simulink library "socmemlib"  (R2021a)
settings: Solver=VariableStepAuto  StartTime=0.0  StopTime=10.0  RelTol=1e-3
PreLoadFcn:
  | soc.internal.HWSWMessageTypeDef();
  | hsb.blkcb2.defineTypes;
undefined symbols (not defined in the file or in its folder): BurstRequest2BusObj, gcbh, hsb, m, ReadAccessBusObj, rearb, RegA, sendFifoFreeMsg, soc, WriteAccessBusObj
libraries: socmemlib_internal x59, priv_hsblib_beta2 x34, socsharedlib_internal x2, socqueuelib_internal x1, simulink x1
(part 3 of 5)

== system socmemlib/IP Core Register Read/Variant/SIM ==
  Wireless Read : socqueuelib_internal/Wireless Read  RegisterName=RegA  DataTypeStr=uint16  Dimensions=1  HoldOutput=on  SampleTime=SampleTime
      settings: SourceProductBaseCode=HW
  " Data" : Outport  VectorParamsAs1DForOutWhenUnconnected=off
  wires:
  Wireless Read/1 -> " Data"/1

== system socmemlib/Memory Channel/Reader 1/From Memory Channel ==
  "readResult " : Inport
  "ctrlIn " : Inport  Port=2
  memReady : Inport  Port=3
  Addressable From Memory Channel : Subsystem  VariantControl=AddressableFromMemory_Variant  mask{PipelineDepth=4, InterconnectDepth=ChTLASTCount}
      mask prompts: PipelineDepth "Read pipeline depth:"; InterconnectDepth "Interconnect queue depth:"
  Software Streaming From Memory Channel : Subsystem  VariantControl=SoftwareStreamingFromMemory_Variant  mask{ReadEventID=BufferEventID, ReadEventVal=[0  0  0  0  0  0  0  0  0  0  0  0  0  0  0  0  0  0  0  0  0  0  0  0  0  0  0  0  0  0  0  0  0  0  0  0  0  0  0  0  0  0  0  0  0  0  0  0  0  0  0  0  0  0  0  0  0  0  0  0  0  0  0  0]}
      mask prompts: ReadEventID "Read event ID"; ReadEventVal "(read event val)"
  Streaming From Memory Channel : Subsystem  VariantControl=StreamingFromMemory_Variant
  Streaming Video From Memory Channel : Subsystem  VariantControl=StreamingVideoFromMemory_Variant
  Streaming Video From Memory Channel with Fsync : Subsystem  VariantControl=StreamingVideoFromMemoryWithFsync_Variant
  " readFromMem" : Outport  VectorParamsAs1DForOutWhenUnconnected=off
  " data" : Outport  Port=2  VectorParamsAs1DForOutWhenUnconnected=off
  " ctrlOut" : Outport  Port=3  VectorParamsAs1DForOutWhenUnconnected=off

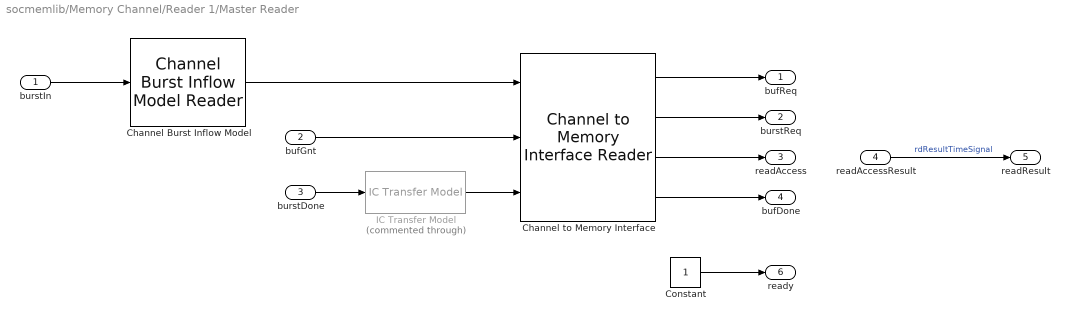
== system socmemlib/Memory Channel/Reader 1/Master Reader ==
  burstIn : Inport
  bufGnt : Inport  Port=2
  burstDone : Inport  Port=3
  readAccessResult : Inport  Port=4
  Channel Burst Inflow Model : priv_hsblib_beta2/Channel Burst Inflow Model Reader  BurstInflowQueueCapacity=EntityInflowQueueCapacity  BurstInflowMeteringTime=EntityInflowTime  MasterKind=MasterKind
      settings: SourceProductBaseCode=HW
  Channel to Memory Interface : priv_hsblib_beta2/Channel to Memory Interface Reader  AccessTransactionType=AccessTransactionType  BufferLengthInBursts=BufferLengthInBursts  MasterKindInt=MasterKind  ICPortNumInt=99
      settings: SourceProductBaseCode=HW
  Constant : Constant  OutDataTypeStr=boolean
  IC Transfer Model : priv_hsblib_beta2/IC Transfer Model  Commented=through  ICFrequency=ICClockFrequency  ICWidth=ICDataWidth
      settings: SourceProductBaseCode=HW
  bufReq : Outport  VectorParamsAs1DForOutWhenUnconnected=off
  burstReq : Outport  Port=2  VectorParamsAs1DForOutWhenUnconnected=off
  readAccess : Outport  Port=3  VectorParamsAs1DForOutWhenUnconnected=off
  bufDone : Outport  Port=4  VectorParamsAs1DForOutWhenUnconnected=off
  readResult : Outport  Port=5  VectorParamsAs1DForOutWhenUnconnected=off
  ready : Outport  Port=6  VectorParamsAs1DForOutWhenUnconnected=off
  wires:
  Channel to Memory Interface/3 -> readAccess/1
  burstDone/1 -> IC Transfer Model/1
  readAccessResult/1 -> readResult/1  "rdResultTimeSignal"
  Channel to Memory Interface/2 -> burstReq/1
  Channel to Memory Interface/1 -> bufReq/1
  burstIn/1 -> Channel Burst Inflow Model/1
  Channel to Memory Interface/4 -> bufDone/1
  bufGnt/1 -> Channel to Memory Interface/2
  Constant/1 -> ready/1
  IC Transfer Model/1 -> Channel to Memory Interface/3
  Channel Burst Inflow Model/1 -> Channel to Memory Interface/1

== system socmemlib/Memory Channel/Reader 1/bufDoneGate ==
  "bufDoneIn " : Inport
  "ctrlIn " : Inport  Port=2
  async : Subsystem  VariantControl=async
  passthrough : Subsystem  VariantControl=passthrough
  " bufDoneOut" : Outport  VectorParamsAs1DForOutWhenUnconnected=off
  " ctrlOut" : Outport  Port=2  VectorParamsAs1DForOutWhenUnconnected=off

== system socmemlib/Memory Channel/Writer 1/Master Writer ==
  note: In this model a new burst request is not made until a burstDone comes back.
      | This means that IC transfers and DDR transfers will be serialized. To get
      | full rate means increasing your IC BW by required DDR BW.
  burstIn : Inport
  bufGnt : Inport  Port=2
  burstDone : Inport  Port=3
  Channel Burst Inflow Model : priv_hsblib_beta2/Channel Burst Inflow Model Writer  BurstInflowQueueCapacity=EntityInflowQueueCapacity  BurstInflowMeteringTime=EntityInflowTime  MasterKind=MasterKind
      settings: SourceProductBaseCode=HW
  Channel to Memory Interface : priv_hsblib_beta2/Channel to Memory Interface Writer  AccessTransactionType=AccessTransactionType  BufferLengthInBursts=BufferLengthInBursts  MasterKindInt=MasterKind  ICPortNumInt=99  FIFODepth=FIFODepth  FIFOAFullDepth=FIFOAFullDepth
      settings: SourceProductBaseCode=HW
  IC Transfer Model : priv_hsblib_beta2/IC Transfer Model  Commented=through  ICFrequency=ICClockFrequency  ICWidth=ICDataWidth
      settings: SourceProductBaseCode=HW
  bufReq : Outport  VectorParamsAs1DForOutWhenUnconnected=off
  burstReq : Outport  Port=2  VectorParamsAs1DForOutWhenUnconnected=off
  wrAccess : Outport  Port=3  VectorParamsAs1DForOutWhenUnconnected=off
  bufDone : Outport  Port=4  VectorParamsAs1DForOutWhenUnconnected=off
  memReady : Outport  Port=5  VectorParamsAs1DForOutWhenUnconnected=off
  wires:
  Channel to Memory Interface/5 -> memReady/1
  IC Transfer Model/1 -> burstReq/1
  burstIn/1 -> Channel Burst Inflow Model/1
  Channel to Memory Interface/4 -> bufDone/1
  Channel to Memory Interface/1 -> bufReq/1
  Channel to Memory Interface/3 -> wrAccess/1
  bufGnt/1 -> Channel to Memory Interface/2
  burstDone/1 -> Channel to Memory Interface/3
  Channel Burst Inflow Model/1 -> Channel to Memory Interface/1
  Channel to Memory Interface/2 -> IC Transfer Model/1

== system socmemlib/Memory Channel/Writer 1/To Memory Channel ==
  "data " : Inport
  "ctrlIn " : Inport  Port=2
  memReady : Inport  Port=3
  Addressable To Memory Channel : Subsystem  VariantControl=AddressableToMemory_Variant  mask{PipelineDepth=16, InterconnectDepth=ChTLASTCount}
      mask prompts: PipelineDepth "Write pipeline depth:"; InterconnectDepth "Interconnect queue depth:"
  Software Streaming To Memory Channel : Subsystem  VariantControl=SoftwareStreamingToMemory_Variant  mask{RequestEventID=BufferEventID, RequestEventVal=[0  0  0  0  0  0  0  0  0  0  0  0  0  0  0  0  0  0  0  0  0  0  0  0  0  0  0  0  0  0  0  0  0  0  0  0  0  0  0  0  0  0  0  0  0  0  0  0  0  0  0  0  0  0  0  0  0  0  0  0  0  0  0  0]}
      mask prompts: RequestEventID "Request event ID"; RequestEventVal "(request event val)"
  Streaming To Memory Channel : Subsystem  VariantControl=StreamingToMemory_Variant
  Streaming Video To Memory Channel : Subsystem  VariantControl=StreamingVideoToMemory_Variant
  " writeToMem" : Outport  VectorParamsAs1DForOutWhenUnconnected=off
  " ctrlOut" : Outport  Port=2  VectorParamsAs1DForOutWhenUnconnected=off
  wrDone : Outport  Port=3

== system socmemlib/Memory Channel/Writer 1/bufDoneGate ==
  "BufDoneIn " : Inport
  "DoneIn " : Inport  Port=2
  async : Subsystem  VariantControl=async
  passthrough : Subsystem  VariantControl=passthrough
  " BufDoneOut" : Outport  VectorParamsAs1DForOutWhenUnconnected=off
  " DoneOut" : Outport  Port=2  VectorParamsAs1DForOutWhenUnconnected=off

== system socmemlib/Memory Channel/Writer 1/bufReqGate ==
  "BufGntIn " : Inport
  "ctrlIn " : Inport  Port=2
  async : Subsystem  VariantControl=async
  passthrough : Subsystem  VariantControl=passthrough
  " BufGntOut" : Outport  VectorParamsAs1DForOutWhenUnconnected=off
  " ctrlOut" : Outport  Port=2  VectorParamsAs1DForOutWhenUnconnected=off

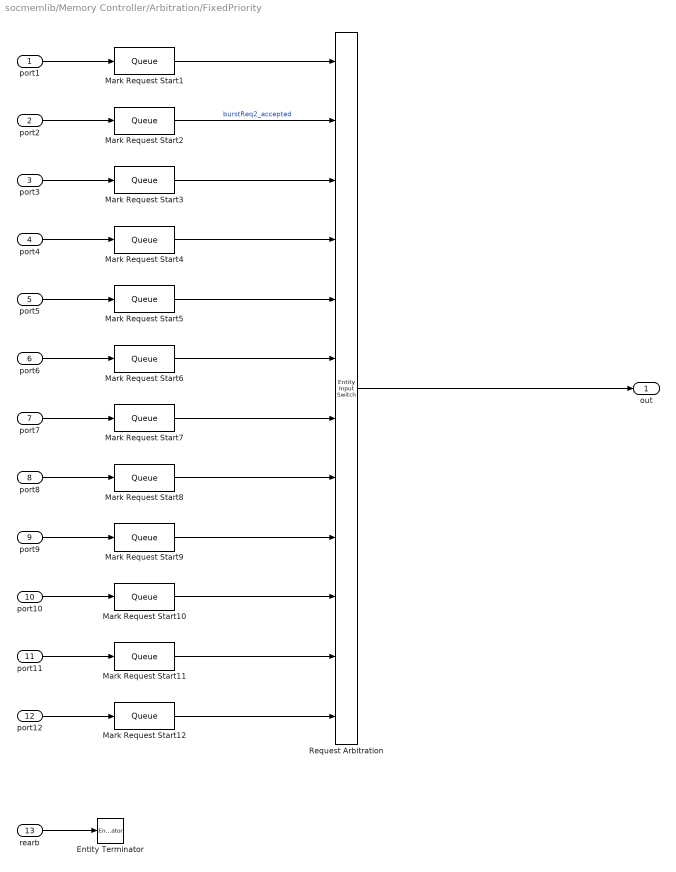
== system socmemlib/Memory Controller/Arbitration/FixedPriority ==
  "port1 " : Inport
  port2 : Inport  Port=2
  port3 : Inport  Port=3
  port4 : Inport  Port=4
  port5 : Inport  Port=5
  port6 : Inport  Port=6
  port7 : Inport  Port=7
  port8 : Inport  Port=8
  port9 : Inport  Port=9
  port10 : Inport  Port=10
  port11 : Inport  Port=11
  port12 : Inport  Port=12
  rearb : Inport  Port=13
  Entity Terminator : EntityTerminator  InputPortMessageModes=m
  Mark Request Start1 : Queue  InputPortMessageModes=m  OutputPortMessageModes=m  Capacity=1  ExitAction=|
      | ddinfo = [entity.masterID; entity.reqID; entity.size; entity.addr; 0];
      | ddlogger(entity.port, DDEvent2.BurstAccepted, ddinfo);
      settings: AttributesFormatString=Capacity=%<Capacity>
  Mark Request Start10 : Queue  InputPortMessageModes=m  OutputPortMessageModes=m  Capacity=1  ExitAction=|
      | ddinfo = [entity.masterID; entity.reqID; entity.size; entity.addr; 0];
      | ddlogger(entity.port, DDEvent2.BurstAccepted, ddinfo);
      settings: AttributesFormatString=Capacity=%<Capacity>
  Mark Request Start11 : Queue  InputPortMessageModes=m  OutputPortMessageModes=m  Capacity=1  ExitAction=|
      | ddinfo = [entity.masterID; entity.reqID; entity.size; entity.addr; 0];
      | ddlogger(entity.port, DDEvent2.BurstAccepted, ddinfo);
      settings: AttributesFormatString=Capacity=%<Capacity>
  Mark Request Start12 : Queue  InputPortMessageModes=m  OutputPortMessageModes=m  Capacity=1  ExitAction=|
      | ddinfo = [entity.masterID; entity.reqID; entity.size; entity.addr; 0];
      | ddlogger(entity.port, DDEvent2.BurstAccepted, ddinfo);
      settings: AttributesFormatString=Capacity=%<Capacity>
  Mark Request Start2 : Queue  InputPortMessageModes=m  OutputPortMessageModes=m  Capacity=1  ExitAction=|
      | ddinfo = [entity.masterID; entity.reqID; entity.size; entity.addr; 0];
      | ddlogger(entity.port, DDEvent2.BurstAccepted, ddinfo);
      settings: AttributesFormatString=Capacity=%<Capacity>
  Mark Request Start3 : Queue  InputPortMessageModes=m  OutputPortMessageModes=m  Capacity=1  ExitAction=|
      | ddinfo = [entity.masterID; entity.reqID; entity.size; entity.addr; 0];
      | ddlogger(entity.port, DDEvent2.BurstAccepted, ddinfo);
      settings: AttributesFormatString=Capacity=%<Capacity>
  Mark Request Start4 : Queue  InputPortMessageModes=m  OutputPortMessageModes=m  Capacity=1  ExitAction=|
      | ddinfo = [entity.masterID; entity.reqID; entity.size; entity.addr; 0];
      | ddlogger(entity.port, DDEvent2.BurstAccepted, ddinfo);
      settings: AttributesFormatString=Capacity=%<Capacity>
  Mark Request Start5 : Queue  InputPortMessageModes=m  OutputPortMessageModes=m  Capacity=1  ExitAction=|
      | ddinfo = [entity.masterID; entity.reqID; entity.size; entity.addr; 0];
      | ddlogger(entity.port, DDEvent2.BurstAccepted, ddinfo);
      settings: AttributesFormatString=Capacity=%<Capacity>
  Mark Request Start6 : Queue  InputPortMessageModes=m  OutputPortMessageModes=m  Capacity=1  ExitAction=|
      | ddinfo = [entity.masterID; entity.reqID; entity.size; entity.addr; 0];
      | ddlogger(entity.port, DDEvent2.BurstAccepted, ddinfo);
      settings: AttributesFormatString=Capacity=%<Capacity>
  Mark Request Start7 : Queue  InputPortMessageModes=m  OutputPortMessageModes=m  Capacity=1  ExitAction=|
      | ddinfo = [entity.masterID; entity.reqID; entity.size; entity.addr; 0];
      | ddlogger(entity.port, DDEvent2.BurstAccepted, ddinfo);
      settings: AttributesFormatString=Capacity=%<Capacity>
  Mark Request Start8 : Queue  InputPortMessageModes=m  OutputPortMessageModes=m  Capacity=1  ExitAction=|
      | ddinfo = [entity.masterID; entity.reqID; entity.size; entity.addr; 0];
      | ddlogger(entity.port, DDEvent2.BurstAccepted, ddinfo);
      settings: AttributesFormatString=Capacity=%<Capacity>
  Mark Request Start9 : Queue  InputPortMessageModes=m  OutputPortMessageModes=m  Capacity=1  ExitAction=|
      | ddinfo = [entity.masterID; entity.reqID; entity.size; entity.addr; 0];
      | ddlogger(entity.port, DDEvent2.BurstAccepted, ddinfo);
      settings: AttributesFormatString=Capacity=%<Capacity>
  Request Arbitration : EntityInputSwitch  InputPortMessageModes=m,m,m,m,m,m,m,m,m,m,m,m  OutputPortMessageModes=m  NumberInputPorts=MAX_NUM_MASTERS
      settings: AttributesFormatString=Criterion=%<SwitchingCriterion>  InputPortMap=u1,u2,u3,u4,u5,u6,u7,u8,u9,u10,u11,u12
  out : Outport  VectorParamsAs1DForOutWhenUnconnected=off
  wires:
  port12/1 -> Mark Request Start12/1
  Mark Request Start12/1 -> Request Arbitration/12
  port11/1 -> Mark Request Start11/1
  Mark Request Start11/1 -> Request Arbitration/11
  port10/1 -> Mark Request Start10/1
  Mark Request Start10/1 -> Request Arbitration/10
  port9/1 -> Mark Request Start9/1
  Mark Request Start9/1 -> Request Arbitration/9
  rearb/1 -> Entity Terminator/1
  Mark Request Start5/1 -> Request Arbitration/5
  Mark Request Start1/1 -> Request Arbitration/1
  Mark Request Start7/1 -> Request Arbitration/7
  port6/1 -> Mark Request Start6/1
  Mark Request Start6/1 -> Request Arbitration/6
  port2/1 -> Mark Request Start2/1
  port7/1 -> Mark Request Start7/1
  Mark Request Start3/1 -> Request Arbitration/3
  "port1 "/1 -> Mark Request Start1/1
  Mark Request Start8/1 -> Request Arbitration/8
  port8/1 -> Mark Request Start8/1
  Request Arbitration/1 -> out/1
  port3/1 -> Mark Request Start3/1
  Mark Request Start4/1 -> Request Arbitration/4
  port4/1 -> Mark Request Start4/1
  port5/1 -> Mark Request Start5/1
  Mark Request Start2/1 -> Request Arbitration/2  "burstReq2_accepted"

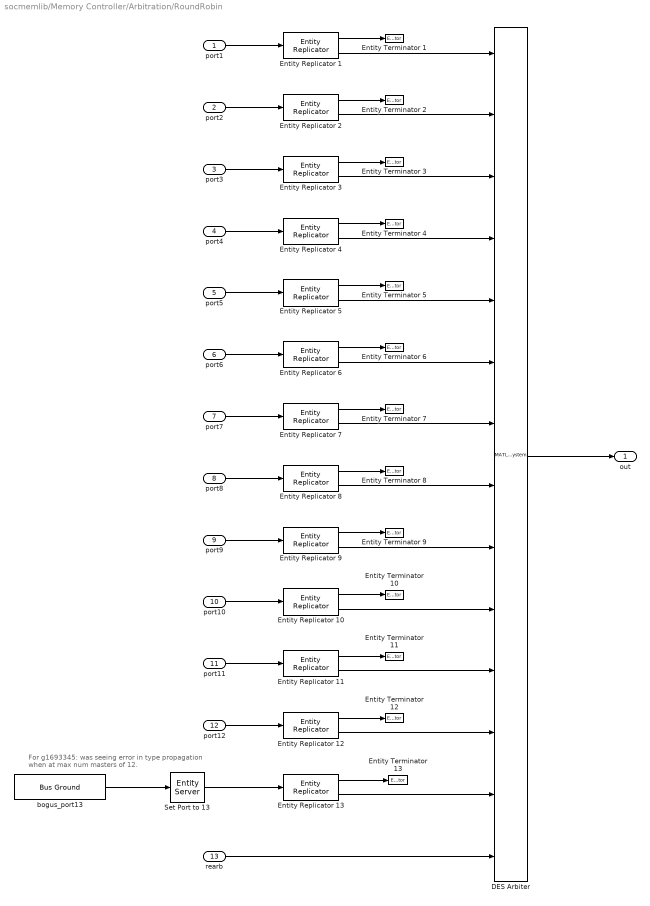
== system socmemlib/Memory Controller/Arbitration/RoundRobin ==
  note: For g1693345: was seeing error in type propagation
      | when at max num masters of 12.
  port1 : Inport
  port2 : Inport  Port=2
  port3 : Inport  Port=3
  port4 : Inport  Port=4
  port5 : Inport  Port=5
  port6 : Inport  Port=6
  port7 : Inport  Port=7
  port8 : Inport  Port=8
  port9 : Inport  Port=9
  port10 : Inport  Port=10
  port11 : Inport  Port=11
  port12 : Inport  Port=12
  rearb : Inport  Port=13
  DES Arbiter : MATLABDiscreteEventSystem  InputPortMessageModes=m,m,m,m,m,m,m,m,m,m,m,m,m,m  OutputPortMessageModes=m  System=hsb.blkcb2.MemoryInterconnectArbitration  NumMasters=MAX_NUM_MASTERS+1  Policy=Round robin  ArbDelay=1e-9  SimulateUsing=Code generation
      mask Type: hsb.blkcb2.MemoryInterconnectArbitration
      mask Display: disp('MemoryInterconnectArbitration');
  Entity Replicator {1..13} (13 alike) : EntityReplicator  InputPortMessageModes=m  OutputPortMessageModes=m,m  HoldOriginalEntityUntilAllReplicasDepart=on
  Entity Terminator 1 : EntityTerminator  InputPortMessageModes=m  EntryAction=|
      | ddinfo = [entity.masterID; entity.reqID; entity.size; entity.addr; 0];
      | ddlogger(entity.port, DDEvent2.BurstAccepted, ddinfo);
  Entity Terminator 10 : EntityTerminator  InputPortMessageModes=m  EntryAction=|
      | ddinfo = [entity.masterID; entity.reqID; entity.size; entity.addr; 0];
      | ddlogger(entity.port, DDEvent2.BurstAccepted, ddinfo);
  Entity Terminator 11 : EntityTerminator  InputPortMessageModes=m  EntryAction=|
      | ddinfo = [entity.masterID; entity.reqID; entity.size; entity.addr; 0];
      | ddlogger(entity.port, DDEvent2.BurstAccepted, ddinfo);
  Entity Terminator 12 : EntityTerminator  InputPortMessageModes=m  EntryAction=|
      | ddinfo = [entity.masterID; entity.reqID; entity.size; entity.addr; 0];
      | ddlogger(entity.port, DDEvent2.BurstAccepted, ddinfo);
  Entity Terminator 13 : EntityTerminator  InputPortMessageModes=m
  Entity Terminator 2 : EntityTerminator  InputPortMessageModes=m  EntryAction=|
      | ddinfo = [entity.masterID; entity.reqID; entity.size; entity.addr; 0];
      | ddlogger(entity.port, DDEvent2.BurstAccepted, ddinfo);
  Entity Terminator 3 : EntityTerminator  InputPortMessageModes=m  EntryAction=|
      | ddinfo = [entity.masterID; entity.reqID; entity.size; entity.addr; 0];
      | ddlogger(entity.port, DDEvent2.BurstAccepted, ddinfo);
  Entity Terminator 4 : EntityTerminator  InputPortMessageModes=m  EntryAction=|
      | ddinfo = [entity.masterID; entity.reqID; entity.size; entity.addr; 0];
      | ddlogger(entity.port, DDEvent2.BurstAccepted, ddinfo);
  Entity Terminator 5 : EntityTerminator  InputPortMessageModes=m  EntryAction=|
      | ddinfo = [entity.masterID; entity.reqID; entity.size; entity.addr; 0];
      | ddlogger(entity.port, DDEvent2.BurstAccepted, ddinfo);
  Entity Terminator 6 : EntityTerminator  InputPortMessageModes=m  EntryAction=|
      | ddinfo = [entity.masterID; entity.reqID; entity.size; entity.addr; 0];
      | ddlogger(entity.port, DDEvent2.BurstAccepted, ddinfo);
  Entity Terminator 7 : EntityTerminator  InputPortMessageModes=m  EntryAction=|
      | ddinfo = [entity.masterID; entity.reqID; entity.size; entity.addr; 0];
      | ddlogger(entity.port, DDEvent2.BurstAccepted, ddinfo);
  Entity Terminator 8 : EntityTerminator  InputPortMessageModes=m  EntryAction=|
      | ddinfo = [entity.masterID; entity.reqID; entity.size; entity.addr; 0];
      | ddlogger(entity.port, DDEvent2.BurstAccepted, ddinfo);
  Entity Terminator 9 : EntityTerminator  InputPortMessageModes=m  EntryAction=|
      | ddinfo = [entity.masterID; entity.reqID; entity.size; entity.addr; 0];
      | ddlogger(entity.port, DDEvent2.BurstAccepted, ddinfo);
  Set Port to 13 : EntityServer  InputPortMessageModes=m  OutputPortMessageModes=m  Capacity=1  ServiceTimeValue=0  EntryAction=|
      | entity.port = 13;
      | entity.state = DDEvent2.BurstRequest;
  bogus_port13 : socmemlib_internal/Bus Ground  OutDataTypeStr=Bus: BurstRequest2BusObj
      settings: SourceProductBaseCode=HW
  out : Outport  VectorParamsAs1DForOutWhenUnconnected=off
  wires:
  Entity Replicator 13/2 -> DES Arbiter/13
  Entity Replicator 13/1 -> Entity Terminator 13/1
  Set Port to 13/1 -> Entity Replicator 13/1
  bogus_port13/1 -> Set Port to 13/1
  Entity Replicator 12/1 -> Entity Terminator 12/1
  port12/1 -> Entity Replicator 12/1
  Entity Replicator 12/2 -> DES Arbiter/12
  Entity Replicator 11/1 -> Entity Terminator 11/1
  port11/1 -> Entity Replicator 11/1
  Entity Replicator 11/2 -> DES Arbiter/11
  Entity Replicator 10/1 -> Entity Terminator 10/1
  port10/1 -> Entity Replicator 10/1
  Entity Replicator 10/2 -> DES Arbiter/10
  Entity Replicator 9/1 -> Entity Terminator 9/1
  port9/1 -> Entity Replicator 9/1
  Entity Replicator 9/2 -> DES Arbiter/9
  Entity Replicator 8/2 -> DES Arbiter/8
  Entity Replicator 7/2 -> DES Arbiter/7
  Entity Replicator 1/2 -> DES Arbiter/1
  Entity Replicator 6/2 -> DES Arbiter/6
  Entity Replicator 2/2 -> DES Arbiter/2
  Entity Replicator 5/2 -> DES Arbiter/5
  Entity Replicator 3/2 -> DES Arbiter/3
  Entity Replicator 4/2 -> DES Arbiter/4
  rearb/1 -> DES Arbiter/14
  port8/1 -> Entity Replicator 8/1
  Entity Replicator 8/1 -> Entity Terminator 8/1
  port7/1 -> Entity Replicator 7/1
  Entity Replicator 7/1 -> Entity Terminator 7/1
  port6/1 -> Entity Replicator 6/1
  Entity Replicator 6/1 -> Entity Terminator 6/1
  port5/1 -> Entity Replicator 5/1
  Entity Replicator 5/1 -> Entity Terminator 5/1
  port4/1 -> Entity Replicator 4/1
  Entity Replicator 4/1 -> Entity Terminator 4/1
  port3/1 -> Entity Replicator 3/1
  Entity Replicator 3/1 -> Entity Terminator 3/1
  port2/1 -> Entity Replicator 2/1
  Entity Replicator 2/1 -> Entity Terminator 2/1
  port1/1 -> Entity Replicator 1/1
  Entity Replicator 1/1 -> Entity Terminator 1/1
  DES Arbiter/1 -> out/1

== system socmemlib/Memory Traffic Generator/Request Queue with Drops/FIFO with Drops ==
  transactionIn : Inport
  Downstream Ready FIFO : Queue  InputPortMessageModes=m  OutputPortMessageModes=m  Capacity=1  ExitAction=sendFifoFreeMsg();
  FIFO with Drops : Stateflow chart  TreatAsAtomicUnit=on
  Simulink Function : Subsystem  TreatAsAtomicUnit=on
  transactionOut : Outport  VectorParamsAs1DForOutWhenUnconnected=off
  fifoStatusMsg : Outport  Port=2  VectorParamsAs1DForOutWhenUnconnected=off
  wires:
  transactionIn/1 -> FIFO with Drops/1(transactionIn)
  Simulink Function/1(Out1) -> FIFO with Drops/2(downstreamEmpty)  "downMsg"
  Downstream Ready FIFO/1 -> transactionOut/1  "postDropFIFO"
  FIFO with Drops/2(fifoStatusMsg) -> fifoStatusMsg/1  "fifoStatusEntity"
  FIFO with Drops/1(transactionOut) -> Downstream Ready FIFO/1

== system socmemlib/Memory Traffic Generator/Request Queue with Drops/Simulink Function ==
  extractOverflow : TriggerPort  TriggerType=function-call  IsSimulinkFunction=on  FunctionName=extractOverflow  FunctionVisibility=scoped  VariantControl=(inherit)
  o : ArgIn  DisableCoverage=on  ArgumentName=o
  overrun : Outport  VectorParamsAs1DForOutWhenUnconnected=off
  wires:
  o/1 -> overrun/1

== system socmemlib/Memory Channel/Reader 1/From Memory Channel/Addressable From Memory Channel ==
  readResult : Inport
  ctrlIn : Inport  Port=2
  memReady : Inport  Port=3
  Addressable Channel Read Slave Interface : Subsystem
  Unit Delay : UnitDelay  SampleTime=-1  HasFrameUpgradeWarning=on
  readFromMem : Outport  VectorParamsAs1DForOutWhenUnconnected=off
  data : Outport  Port=2  VectorParamsAs1DForOutWhenUnconnected=off
  ctrlOut : Outport  Port=3  VectorParamsAs1DForOutWhenUnconnected=off
  wires:
  Unit Delay/1 -> Addressable Channel Read Slave Interface/2(rdCtrlM2S)
  Addressable Channel Read Slave Interface/2(dataOut) -> data/1
  memReady/1 -> Addressable Channel Read Slave Interface/3(memReady)
  Addressable Channel Read Slave Interface/1(readFromMem) -> readFromMem/1
  Addressable Channel Read Slave Interface/3(rdCtrlS2M) -> ctrlOut/1
  ctrlIn/1 -> Unit Delay/1
  readResult/1 -> Addressable Channel Read Slave Interface/1(rdResult)

== system socmemlib/Memory Channel/Reader 1/From Memory Channel/Software Streaming From Memory Channel ==
  readResult : Inport
  ctrlIn : Inport  Port=2
  memReady : Inport  Port=3
  Channel Streaming Master Interface : Subsystem
  readFromMem : Outport  VectorParamsAs1DForOutWhenUnconnected=off
  data : Outport  Port=2  VectorParamsAs1DForOutWhenUnconnected=off
  ctrlOut : Outport  Port=3  VectorParamsAs1DForOutWhenUnconnected=off
  wires:
  readResult/1 -> Channel Streaming Master Interface/1(rdResult)
  ctrlIn/1 -> Channel Streaming Master Interface/2(ctrlIn)
  Channel Streaming Master Interface/1(readFromMem) -> readFromMem/1
  memReady/1 -> Channel Streaming Master Interface/3(memReady)
  Channel Streaming Master Interface/2(data) -> data/1
  Channel Streaming Master Interface/3(ctrlOut) -> ctrlOut/1

== system socmemlib/Memory Channel/Reader 1/From Memory Channel/Streaming From Memory Channel ==
  readResult : Inport
  "ctrlIn " : Inport  Port=2
  memReady : Inport  Port=3
  Bus Selector1 : BusSelector  OutputSignals=ready
  Channel Streaming Master Interface : Subsystem
  Unit Delay : UnitDelay  SampleTime=-1  HasFrameUpgradeWarning=on
  readFromMem : Outport  VectorParamsAs1DForOutWhenUnconnected=off
  data : Outport  Port=2  VectorParamsAs1DForOutWhenUnconnected=off
  " ctrlOut" : Outport  Port=3  VectorParamsAs1DForOutWhenUnconnected=off
  wires:
  Unit Delay/1 -> Channel Streaming Master Interface/1(ready)
  Channel Streaming Master Interface/3(rdCtrlM2S) -> " ctrlOut"/1
  readResult/1 -> Channel Streaming Master Interface/2(rdResult)
  Channel Streaming Master Interface/2(dataOut) -> data/1
  memReady/1 -> Channel Streaming Master Interface/3(memReady)
  Channel Streaming Master Interface/1(readFromMem) -> readFromMem/1
  Bus Selector1/1 -> Unit Delay/1  "<ready>"
  "ctrlIn "/1 -> Bus Selector1/1

== system socmemlib/Memory Channel/Reader 1/From Memory Channel/Streaming Video From Memory Channel ==
  readResult : Inport
  "ctrlIn " : Inport  Port=2
  memReady : Inport  Port=3
  Bus Selector1 : BusSelector  OutputSignals=ready
  Channel Streaming Master Interface : Subsystem
  Unit Delay : UnitDelay  SampleTime=-1  HasFrameUpgradeWarning=on
  readFromMem : Outport  VectorParamsAs1DForOutWhenUnconnected=off
  data : Outport  Port=2  VectorParamsAs1DForOutWhenUnconnected=off
  " ctrlOut" : Outport  Port=3  VectorParamsAs1DForOutWhenUnconnected=off
  wires:
  Unit Delay/1 -> Channel Streaming Master Interface/1(ready)
  readResult/1 -> Channel Streaming Master Interface/2(rdResult)
  Channel Streaming Master Interface/2(pixel) -> data/1
  memReady/1 -> Channel Streaming Master Interface/3(memReady)
  Channel Streaming Master Interface/1(readFromMem) -> readFromMem/1
  Channel Streaming Master Interface/3(ctrl) -> " ctrlOut"/1
  "ctrlIn "/1 -> Bus Selector1/1
  Bus Selector1/1 -> Unit Delay/1  "<ready>"

== system socmemlib/Memory Channel/Reader 1/From Memory Channel/Streaming Video From Memory Channel with Fsync ==
  readResult : Inport
  "ctrlIn " : Inport  Port=2
  memReady : Inport  Port=3
  Bus Selector1 : BusSelector  OutputSignals=ready,fsync
  Channel Streaming Master Interface : Subsystem
  From Frame Buffer Interface : Subsystem  InitFcn=hsb.blkcb2.defineTypes;
  readFromMem : Outport  VectorParamsAs1DForOutWhenUnconnected=off
  data : Outport  Port=2  VectorParamsAs1DForOutWhenUnconnected=off
  " ctrlOut" : Outport  Port=3  VectorParamsAs1DForOutWhenUnconnected=off
  wires:
  Bus Selector1/2 -> From Frame Buffer Interface/2(frameSync)  "<fsync>"
  readResult/1 -> Channel Streaming Master Interface/2(rdResult)
  Channel Streaming Master Interface/2(pixel) -> data/1
  memReady/1 -> Channel Streaming Master Interface/3(memReady)
  Channel Streaming Master Interface/1(readFromMem) -> readFromMem/1
  Channel Streaming Master Interface/3(ctrl) -> " ctrlOut"/1
  "ctrlIn "/1 -> Bus Selector1/1
  From Frame Buffer Interface/1(rdyToUp) -> Channel Streaming Master Interface/1(ready)
  Bus Selector1/1 -> From Frame Buffer Interface/1(rdyFromDown)  "<ready>"

== system socmemlib/Memory Channel/Reader 1/bufDoneGate/async ==
  bufDoneIn : Inport
  ctrlIn : Inport  Port=2
  Buffer Release Gate : Stateflow chart  TreatAsAtomicUnit=on
  Entity Replicator : EntityReplicator  InputPortMessageModes=m  OutputPortMessageModes=m,m
  bufDoneOut : Outport  VectorParamsAs1DForOutWhenUnconnected=off
  ctrlOut : Outport  Port=2  VectorParamsAs1DForOutWhenUnconnected=off
  wires:
  ctrlIn/1 -> Entity Replicator/1
  Entity Replicator/2 -> ctrlOut/1
  Entity Replicator/1 -> Buffer Release Gate/2(frameDone)
  Buffer Release Gate/1(bufDoneOut) -> bufDoneOut/1
  bufDoneIn/1 -> Buffer Release Gate/1(bufDoneIn)

== system socmemlib/Memory Channel/Reader 1/bufDoneGate/passthrough ==
  bufDoneIn : Inport
  ctrlIn : Inport  Port=2
  bufDoneOut : Outport  VectorParamsAs1DForOutWhenUnconnected=off
  ctrlOut : Outport  Port=2  VectorParamsAs1DForOutWhenUnconnected=off
  wires:
  ctrlIn/1 -> ctrlOut/1
  bufDoneIn/1 -> bufDoneOut/1

== system socmemlib/Memory Channel/Writer 1/To Memory Channel/Addressable To Memory Channel ==
  data : Inport
  "ctrlIn " : Inport  Port=2
  memReady : Inport  Port=3
  Addressable Channel Write Slave Interface : Subsystem
  Check Signal Attributes : priv_hsblib_beta2/Check Signal Attributes  stime=ChFrameSampleTime  dims=ChDimensions  dtype=ChType  ptype=memory
      settings: SourceProductBaseCode=HW
  writeToMem : Outport  VectorParamsAs1DForOutWhenUnconnected=off
  " ctrlOut" : Outport  Port=2  VectorParamsAs1DForOutWhenUnconnected=off
  wires:
  Addressable Channel Write Slave Interface/2(wrCtrlS2M) -> " ctrlOut"/1
  memReady/1 -> Addressable Channel Write Slave Interface/3(memReady)
  Addressable Channel Write Slave Interface/1(writeToMem) -> writeToMem/1
  data/1 -> Check Signal Attributes/1, Addressable Channel Write Slave Interface/1(dataIn)
  "ctrlIn "/1 -> Addressable Channel Write Slave Interface/2(wrCtrlM2S)

== system socmemlib/Memory Channel/Writer 1/To Memory Channel/Software Streaming To Memory Channel ==
  data : Inport
  ctrlIn : Inport  Port=2
  memReady : Inport  Port=3
  Channel Streaming Slave Interface : Subsystem
  Terminator : Terminator
  Terminator1 : Terminator
  writeToMem : Outport  VectorParamsAs1DForOutWhenUnconnected=off
  ctrlOut : Outport  Port=2  VectorParamsAs1DForOutWhenUnconnected=off
  wrDone : Outport  Port=3
  wires:
  Channel Streaming Slave Interface/3(wrDone) -> wrDone/1
  data/1 -> Channel Streaming Slave Interface/1(data)
  Channel Streaming Slave Interface/2(ctrlOut) -> ctrlOut/1
  memReady/1 -> Terminator1/1
  Channel Streaming Slave Interface/1(writeToMem) -> writeToMem/1
  ctrlIn/1 -> Terminator/1

== system socmemlib/Memory Channel/Writer 1/To Memory Channel/Streaming To Memory Channel ==
  data : Inport
  "ctrlIn " : Inport  Port=2
  memReady : Inport  Port=3
  Bus Creator : BusCreator  Inputs=1  OutDataTypeStr=Bus: StreamS2MBusObj  NonVirtualBus=on
      settings: InheritFromInputs=off
  Bus Selector : BusSelector  OutputSignals=valid,tlast
  Channel Streaming Slave Interface : Subsystem
  Check Signal Attributes : priv_hsblib_beta2/Check Signal Attributes  stime=ChFrameSampleTime  dims=ChDimensions  dtype=ChType  ptype=memory
      settings: SourceProductBaseCode=HW
  writeToMem : Outport  VectorParamsAs1DForOutWhenUnconnected=off
  " ctrlOut" : Outport  Port=2  VectorParamsAs1DForOutWhenUnconnected=off
  wires:
  Bus Creator/1 -> " ctrlOut"/1
  Bus Selector/2 -> Channel Streaming Slave Interface/3(tlast)  "<tlast>"
  Bus Selector/1 -> Channel Streaming Slave Interface/2(valid)  "<valid>"
  memReady/1 -> Channel Streaming Slave Interface/4(memReady)
  Channel Streaming Slave Interface/1(writeToMem) -> writeToMem/1
  data/1 -> Check Signal Attributes/1, Channel Streaming Slave Interface/1(data)
  Channel Streaming Slave Interface/2(ready) -> Bus Creator/1
  "ctrlIn "/1 -> Bus Selector/1

== system socmemlib/Memory Channel/Writer 1/To Memory Channel/Streaming Video To Memory Channel ==
  data : Inport
  "ctrlIn " : Inport  Port=2
  memReady : Inport  Port=3
  Bus Creator : BusCreator  Inputs=1  OutDataTypeStr=Bus: StreamVideoS2MBusObj  NonVirtualBus=on
      settings: InheritFromInputs=off
  Channel Streaming Video Slave Interface : Subsystem
  Check Signal Attributes : priv_hsblib_beta2/Check Signal Attributes  stime=ChFrameSampleTime  dims=ChDimensions  dtype=ChType  ptype=memory
      settings: SourceProductBaseCode=HW
  writeToMem : Outport  VectorParamsAs1DForOutWhenUnconnected=off
  " ctrlOut" : Outport  Port=2  VectorParamsAs1DForOutWhenUnconnected=off
  wires:
  Bus Creator/1 -> " ctrlOut"/1
  memReady/1 -> Channel Streaming Video Slave Interface/3(memReady)
  Channel Streaming Video Slave Interface/1(writeToMem) -> writeToMem/1
  data/1 -> Check Signal Attributes/1, Channel Streaming Video Slave Interface/1(data)
  Channel Streaming Video Slave Interface/2(ready) -> Bus Creator/1
  "ctrlIn "/1 -> Channel Streaming Video Slave Interface/2(pixelcontrol)

== system socmemlib/Memory Channel/Writer 1/bufDoneGate/async ==
  "BufDoneIn " : Inport
  "DoneIn " : Inport  Port=2
  Buffer Request Gate : Stateflow chart  TreatAsAtomicUnit=on
  Entity Queue : Queue  InputPortMessageModes=m  OutputPortMessageModes=m  OverwriteOldest=on  Capacity=MRNumBuffers
  Entity Replicator : EntityReplicator  InputPortMessageModes=m  OutputPortMessageModes=m,m
  " DoneOut" : Outport  VectorParamsAs1DForOutWhenUnconnected=off
  " BufDoneOut" : Outport  Port=2  VectorParamsAs1DForOutWhenUnconnected=off
  wires:
  Entity Queue/1 -> " DoneOut"/1
  Entity Replicator/1 -> Buffer Request Gate/2(BufDoneIn)
  Entity Replicator/2 -> " BufDoneOut"/1
  "BufDoneIn "/1 -> Entity Replicator/1
  Buffer Request Gate/1(DoneOut) -> Entity Queue/1
  "DoneIn "/1 -> Buffer Request Gate/1(DoneIn)

== system socmemlib/Memory Channel/Writer 1/bufDoneGate/passthrough ==
  "BufDoneIn " : Inport
  "DoneIn " : Inport  Port=2
  " BufDoneOut" : Outport  VectorParamsAs1DForOutWhenUnconnected=off
  " DoneOut" : Outport  Port=2  VectorParamsAs1DForOutWhenUnconnected=off
  wires:
  "BufDoneIn "/1 -> " BufDoneOut"/1
  "DoneIn "/1 -> " DoneOut"/1

== system socmemlib/Memory Channel/Writer 1/bufReqGate/async ==
  BufGntIn : Inport
  "ctrlIn " : Inport  Port=2
  Buffer Request Gate : Stateflow chart  TreatAsAtomicUnit=on
  Entity Replicator : EntityReplicator  InputPortMessageModes=m  OutputPortMessageModes=m,m
  BufGntOut : Outport  VectorParamsAs1DForOutWhenUnconnected=off
  ctrlOut : Outport  Port=2  VectorParamsAs1DForOutWhenUnconnected=off
  wires:
  BufGntIn/1 -> Entity Replicator/1
  Entity Replicator/2 -> BufGntOut/1
  Entity Replicator/1 -> Buffer Request Gate/2(BufGntIn)
  Buffer Request Gate/1(bufReqOut) -> ctrlOut/1
  "ctrlIn "/1 -> Buffer Request Gate/1(bufReqIn)

== system socmemlib/Memory Channel/Writer 1/bufReqGate/passthrough ==
  "BufGntIn " : Inport
  ctrlIn : Inport  Port=2
  " BufGntOut" : Outport  VectorParamsAs1DForOutWhenUnconnected=off
  ctrlOut : Outport  Port=2  VectorParamsAs1DForOutWhenUnconnected=off
  wires:
  ctrlIn/1 -> ctrlOut/1
  "BufGntIn "/1 -> " BufGntOut"/1

== system socmemlib/Memory Traffic Generator/Request Queue with Drops/FIFO with Drops/Simulink Function ==
  sendFifoFreeMsg : TriggerPort  TriggerType=function-call  IsSimulinkFunction=on  FunctionName=sendFifoFreeMsg  FunctionVisibility=scoped  VariantControl=Variant
  Constant : Constant
  Message Send : Send  OutputPortMessageModes=m
  Out1 : Outport  VectorParamsAs1DForOutWhenUnconnected=off
  wires:
  Constant/1 -> Message Send/1
  Message Send/1 -> Out1/1

== system socmemlib/Memory Channel/Reader 1/From Memory Channel/Addressable From Memory Channel/Addressable Channel Read Slave Interface ==
  rdResult : Inport
  rdCtrlM2S : Inport  Port=2
  memReady : Inport  Port=3
  A4M Rd Slave BFM : Stateflow chart  TreatAsAtomicUnit=on
  unpackFromBytes : priv_hsblib_beta2/unpackFromBytes  ChDimensions=ChDimensions  ChType=ChType  ChBitPacked=ChBitPacked  ChWidth=ChWidth  ChTDATAWidth=ChTDATAWidth  ChCompLength=ChCompLength  ChCompBitRanges=ChCompBitRanges  ChContainerType=ChContainerType  ChLength=ChLength
      settings: SourceProductBaseCode=HW
  readFromMem : Outport  VectorParamsAs1DForOutWhenUnconnected=off
  dataOut : Outport  Port=2  VectorParamsAs1DForOutWhenUnconnected=off
  rdCtrlS2M : Outport  Port=3  VectorParamsAs1DForOutWhenUnconnected=off
  wires:
  A4M Rd Slave BFM/3(rdCtrlS2M) -> rdCtrlS2M/1
  A4M Rd Slave BFM/2(packDataOut) -> unpackFromBytes/1
  rdCtrlM2S/1 -> A4M Rd Slave BFM/2(rdCtrlM2S)
  rdResult/1 -> A4M Rd Slave BFM/1(rdResult)
  unpackFromBytes/1 -> dataOut/1
  memReady/1 -> A4M Rd Slave BFM/3(memReady)
  A4M Rd Slave BFM/1(readFromMem) -> readFromMem/1  "readFromMem"

== system socmemlib/Memory Channel/Reader 1/From Memory Channel/Software Streaming From Memory Channel/Channel Streaming Master Interface ==
  rdResult : Inport
  ctrlIn : Inport  Port=2
  memReady : Inport  Port=3
  A4S Master BFM : Stateflow chart  TreatAsAtomicUnit=on
  MsgSendCtrl : Subsystem
  Terminator6 : Terminator
  readFromMem : Outport  VectorParamsAs1DForOutWhenUnconnected=off
  data : Outport  Port=2  VectorParamsAs1DForOutWhenUnconnected=off
  ctrlOut : Outport  Port=3  VectorParamsAs1DForOutWhenUnconnected=off
  wires:
  ctrlIn/1 -> MsgSendCtrl/1(Done)
  MsgSendCtrl/1(Event) -> ctrlOut/1
  MsgSendCtrl/2(Msg) -> data/1
  rdResult/1 -> A4S Master BFM/1(rdResult)
  memReady/1 -> Terminator6/1
  A4S Master BFM/1(readFromMem) -> readFromMem/1  "readFromMem"

== system socmemlib/Memory Channel/Reader 1/From Memory Channel/Streaming From Memory Channel/Channel Streaming Master Interface ==
  note: CHECKME: Does S/M need this?
  ready : Inport
  rdResult : Inport  Port=2
  memReady : Inport  Port=3
  A4S Master BFM : Stateflow chart  TreatAsAtomicUnit=on
  Terminator : Terminator
  unpackFromBytes : priv_hsblib_beta2/unpackFromBytes  ChDimensions=ChDimensions  ChType=ChType  ChBitPacked=ChBitPacked  ChWidth=ChWidth  ChTDATAWidth=ChTDATAWidth  ChCompLength=ChCompLength  ChCompBitRanges=ChCompBitRanges  ChContainerType=ChContainerType  ChLength=ChLength
      settings: SourceProductBaseCode=HW
  readFromMem : Outport  VectorParamsAs1DForOutWhenUnconnected=off
  dataOut : Outport  Port=2  VectorParamsAs1DForOutWhenUnconnected=off
  rdCtrlM2S : Outport  Port=3  VectorParamsAs1DForOutWhenUnconnected=off
  wires:
  A4S Master BFM/3(rdCtrlM2S) -> rdCtrlM2S/1
  A4S Master BFM/2(packDataOut) -> unpackFromBytes/1
  ready/1 -> A4S Master BFM/1(ready)
  rdResult/1 -> A4S Master BFM/2(rdResult)
  unpackFromBytes/1 -> dataOut/1
  memReady/1 -> Terminator/1  "fromMemFIFOStatus"
  A4S Master BFM/1(readFromMem) -> readFromMem/1  "readFromMem"

== system socmemlib/Memory Channel/Reader 1/From Memory Channel/Streaming Video From Memory Channel/Channel Streaming Master Interface ==
  ready : Inport
  rdResult : Inport  Port=2
  memReady : Inport  Port=3
  A4S Master BFM : Stateflow chart  TreatAsAtomicUnit=on
  Terminator5 : Terminator
  unpackFromBytes : priv_hsblib_beta2/unpackFromBytes  ChDimensions=ChDimensions  ChType=ChType  ChBitPacked=ChBitPacked  ChWidth=ChWidth  ChTDATAWidth=ChTDATAWidth  ChCompLength=ChCompLength  ChCompBitRanges=ChCompBitRanges  ChContainerType=ChContainerType  ChLength=ChLength
      settings: SourceProductBaseCode=HW
  readFromMem : Outport  VectorParamsAs1DForOutWhenUnconnected=off
  pixel : Outport  Port=2  VectorParamsAs1DForOutWhenUnconnected=off
  ctrl : Outport  Port=3  VectorParamsAs1DForOutWhenUnconnected=off
  wires:
  A4S Master BFM/3(ctrl) -> ctrl/1
  A4S Master BFM/2(packDataOut) -> unpackFromBytes/1
  ready/1 -> A4S Master BFM/1(ready)
  rdResult/1 -> A4S Master BFM/2(rdResult)
  unpackFromBytes/1 -> pixel/1
  memReady/1 -> Terminator5/1
  A4S Master BFM/1(readFromMem) -> readFromMem/1

== system socmemlib/Memory Channel/Reader 1/From Memory Channel/Streaming Video From Memory Channel with Fsync/Channel Streaming Master Interface ==
  ready : Inport
  rdResult : Inport  Port=2
  memReady : Inport  Port=3
  A4S Master BFM : Stateflow chart  TreatAsAtomicUnit=on
  Terminator5 : Terminator
  unpackFromBytes : priv_hsblib_beta2/unpackFromBytes  ChDimensions=ChDimensions  ChType=ChType  ChBitPacked=ChBitPacked  ChWidth=ChWidth  ChTDATAWidth=ChTDATAWidth  ChCompLength=ChCompLength  ChCompBitRanges=ChCompBitRanges  ChContainerType=ChContainerType  ChLength=ChLength
      settings: SourceProductBaseCode=HW
  readFromMem : Outport  VectorParamsAs1DForOutWhenUnconnected=off
  pixel : Outport  Port=2  VectorParamsAs1DForOutWhenUnconnected=off
  ctrl : Outport  Port=3  VectorParamsAs1DForOutWhenUnconnected=off
  wires:
  A4S Master BFM/3(ctrl) -> ctrl/1
  A4S Master BFM/2(packDataOut) -> unpackFromBytes/1
  ready/1 -> A4S Master BFM/1(ready)
  rdResult/1 -> A4S Master BFM/2(rdResult)
  unpackFromBytes/1 -> pixel/1
  memReady/1 -> Terminator5/1
  A4S Master BFM/1(readFromMem) -> readFromMem/1  "readFromMem"

== system socmemlib/Memory Channel/Reader 1/From Memory Channel/Streaming Video From Memory Channel with Fsync/From Frame Buffer Interface ==
  rdyFromDown : Inport
  frameSync : Inport  Port=2
  Delay2 : Delay  DelayLength=1
  Delay4 : Delay  DelayLength=1
  Signal Specification2 : SignalSpecification  Dimensions=1  BusOutputAsStruct=on
  Video FIFO Frame Sync Toggle : Subsystem
  rdyToUp : Outport  VectorParamsAs1DForOutWhenUnconnected=off
  wires:
  Delay4/1 -> Video FIFO Frame Sync Toggle/2(frameSync)
  Delay2/1 -> Video FIFO Frame Sync Toggle/1(readyIn)
  Signal Specification2/1 -> rdyToUp/1
  rdyFromDown/1 -> Delay2/1
  frameSync/1 -> Delay4/1
  Video FIFO Frame Sync Toggle/1(readyOut) -> Signal Specification2/1

== system socmemlib/Memory Channel/Writer 1/To Memory Channel/Addressable To Memory Channel/Addressable Channel Write Slave Interface ==
  dataIn : Inport
  wrCtrlM2S : Inport  Port=2
  memReady : Inport  Port=3
  A4M Wr Slave BFM : Stateflow chart  TreatAsAtomicUnit=on
  Chart : Stateflow chart  TreatAsAtomicUnit=on
  Memory : Memory
  Unit Delay : UnitDelay  SampleTime=-1  HasFrameUpgradeWarning=on
  packToBytes : priv_hsblib_beta2/packToBytes  ChDimensions=ChDimensions  ChType=ChType  ChBitPacked=ChBitPacked  ChWidth=ChWidth  ChTDATAWidth=ChTDATAWidth  ChTDATAPadWidth=ChTDATAPadWidth  ChCompLength=ChCompLength  ChFrameGatherBufferSize=ChFrameGatherBufferSize  ChLength=ChLength
      settings: SourceProductBaseCode=HW
  writeToMem : Outport  VectorParamsAs1DForOutWhenUnconnected=off
  wrCtrlS2M : Outport  Port=2  VectorParamsAs1DForOutWhenUnconnected=off
  wires:
  A4M Wr Slave BFM/1(writeToMem) -> writeToMem/1  "writeToMemIn"
  A4M Wr Slave BFM/2(wrCtrlS2M) -> Unit Delay/1  "ch_ready"
  Unit Delay/1 -> wrCtrlS2M/1
  wrCtrlM2S/1 -> A4M Wr Slave BFM/2(wrCtrlM2S)
  memReady/1 -> Memory/1
  Chart/1(readyDiscrete) -> A4M Wr Slave BFM/3(memReady)  "rdyDiscrete"
  Memory/1 -> Chart/1(readyFiM)
  dataIn/1 -> packToBytes/1
  packToBytes/1 -> A4M Wr Slave BFM/1(packDataIn)

== system socmemlib/Memory Channel/Writer 1/To Memory Channel/Software Streaming To Memory Channel/Channel Streaming Slave Interface ==
  data : Inport
  A4S BFM : Stateflow chart  TreatAsAtomicUnit=on
  Check Signal Attributes : priv_hsblib_beta2/Check Signal Attributes  stime=-1  dims=ChDimensions  dtype=ChType  ptype=memory
      settings: SourceProductBaseCode=HW
  Entity Generator : EntityGenerator  InputPortMessageModes=m  OutputPortMessageModes=m  GenerationMethod=Event-based  TimeSource=Signal port  Period=-1  GenerateAction=|  EntityType=Bus object  EntityTypeName=rteEvent
      | entity.name = [uint16('Dummy'), uint16(nan([1,64 - length('Dummy')]))]';
      | entity.type = uint32(5);
      | entity.index = uint32(0);
      settings: InputPortMap=u0
  Entity Replicator : EntityReplicator  InputPortMessageModes=m  OutputPortMessageModes=m,m
  MsgRecvCtrl : Subsystem  TreatAsAtomicUnit=on
  MsgReqCtrl : Subsystem
  writeToMem : Outport  VectorParamsAs1DForOutWhenUnconnected=off
  ctrlOut : Outport  Port=2  VectorParamsAs1DForOutWhenUnconnected=off
  wrDone : Outport  Port=3
  wires:
  Entity Replicator/1 -> Entity Generator/1
  Entity Generator/1 -> A4S BFM/1(event)
  Entity Replicator/2 -> MsgRecvCtrl/1(Msg)
  data/1 -> Entity Replicator/1
  MsgRecvCtrl/1(data) -> Check Signal Attributes/1
  MsgRecvCtrl/2(Done) -> wrDone/1
  MsgReqCtrl/1(Event) -> ctrlOut/1
  A4S BFM/1(writeToMem) -> writeToMem/1  "writeToMemIn"

== system socmemlib/Memory Channel/Writer 1/To Memory Channel/Streaming To Memory Channel/Channel Streaming Slave Interface ==
  data : Inport
  valid : Inport  Port=2
  tlast : Inport  Port=3
  memReady : Inport  Port=4
  A4S BFM : Stateflow chart  TreatAsAtomicUnit=on
  Chart : Stateflow chart  TreatAsAtomicUnit=on
  Memory : Memory
  packToBytes : priv_hsblib_beta2/packToBytes  ChDimensions=ChDimensions  ChType=ChType  ChBitPacked=ChBitPacked  ChWidth=ChWidth  ChTDATAWidth=ChTDATAWidth  ChTDATAPadWidth=ChTDATAPadWidth  ChCompLength=ChCompLength  ChFrameGatherBufferSize=ChFrameGatherBufferSize  ChLength=ChLength
      settings: SourceProductBaseCode=HW
  writeToMem : Outport  VectorParamsAs1DForOutWhenUnconnected=off
  ready : Outport  Port=2  VectorParamsAs1DForOutWhenUnconnected=off
  wires:
  memReady/1 -> Memory/1
  Chart/1(readyDiscrete) -> ready/1
  A4S BFM/1(writeToMem) -> writeToMem/1  "writeToMemIn"
  tlast/1 -> A4S BFM/3(tlast)
  valid/1 -> A4S BFM/2(valid)
  Memory/1 -> Chart/1(readyFiM)
  data/1 -> packToBytes/1
  packToBytes/1 -> A4S BFM/1(packDataIn)

== system socmemlib/Memory Channel/Writer 1/To Memory Channel/Streaming Video To Memory Channel/Channel Streaming Video Slave Interface ==
  data : Inport
  pixelcontrol : Inport  Port=2
  memReady : Inport  Port=3
  A4SV BFM : Stateflow chart  TreatAsAtomicUnit=on
  Chart : Stateflow chart  TreatAsAtomicUnit=on
  Memory : Memory
  packToBytes : priv_hsblib_beta2/packToBytes  ChDimensions=ChDimensions  ChType=ChType  ChBitPacked=ChBitPacked  ChWidth=ChWidth  ChTDATAWidth=ChTDATAWidth  ChTDATAPadWidth=ChTDATAPadWidth  ChCompLength=ChCompLength  ChFrameGatherBufferSize=ChFrameGatherBufferSize  ChLength=ChLength
      settings: SourceProductBaseCode=HW
  writeToMem : Outport  VectorParamsAs1DForOutWhenUnconnected=off
  ready : Outport  Port=2  VectorParamsAs1DForOutWhenUnconnected=off
  wires:
  A4SV BFM/1(writeToMem) -> writeToMem/1  "writeToMemIn"
  pixelcontrol/1 -> A4SV BFM/2(ctrl)
  memReady/1 -> Memory/1
  Chart/1(readyDiscrete) -> ready/1
  Memory/1 -> Chart/1(readyFiM)
  data/1 -> packToBytes/1
  packToBytes/1 -> A4SV BFM/1(packDataIn)

== system socmemlib/Memory Channel/Reader 1/From Memory Channel/Software Streaming From Memory Channel/Channel Streaming Master Interface/MsgSendCtrl ==
  Done : Inport
  MsgSendCtrl : TriggerPort  TriggerType=function-call  IsSimulinkFunction=on  FunctionName=MsgSendCtrl  FunctionVisibility=scoped  VariantControl=Variant
  Constant : Constant  OutDataTypeStr=boolean  SampleTime=-1
  HWSW Message Send : socsharedlib_internal/HWSW Message Send  QueueLength=NumberOfBuffers  MessageType=Stream  MessageID=HWSWMetadataID.Stream  EnableEventPort=on  EnableDonePort=on
      settings: SourceProductBaseCode=HW
  Terminator2 : Terminator
  Width : Width  DataType=uint32
  unpackFromBytes : priv_hsblib_beta2/unpackFromBytes  ChDimensions=ChDimensions  ChType=ChType  ChBitPacked=ChBitPacked  ChWidth=ChWidth  ChTDATAWidth=ChTDATAWidth  ChCompLength=ChCompLength  ChCompBitRanges=ChCompBitRanges  ChContainerType=ChContainerType  ChLength=ChLength
      settings: SourceProductBaseCode=HW
  cmd : ArgIn  OutDataTypeStr=uint8  PortDimensions=ChFrameGatherBufferSize  ArgumentName=Data
  Event : Outport  VectorParamsAs1DForOutWhenUnconnected=off
  Msg : Outport  Port=2  VectorParamsAs1DForOutWhenUnconnected=off
  wires:
  Done/1 -> HWSW Message Send/4
  cmd/1 -> unpackFromBytes/1
  Width/1 -> HWSW Message Send/2
  HWSW Message Send/1 -> Event/1
  Constant/1 -> HWSW Message Send/3
  HWSW Message Send/3 -> Terminator2/1
  HWSW Message Send/2 -> Msg/1
  unpackFromBytes/1 -> Width/1, HWSW Message Send/1  "readFromMem"

== system socmemlib/Memory Channel/Reader 1/From Memory Channel/Streaming Video From Memory Channel with Fsync/From Frame Buffer Interface/Video FIFO Frame Sync Toggle ==
  readyIn : Inport
  frameSync : Inport  Port=2
  Constant : Constant  VectorParams1D=off  OutDataTypeStr=boolean  SampleTime=-1
  Delay : Delay  DelayLength=1  InitialCondition=0  ShowEnablePort=on  UseCircularBuffer=on
      settings: InputPortMap=u0,e6
  Logical Operator : Logic  AllPortsSameDT=off  OutDataTypeStr=boolean
  State Control : StateControl  StateControl=Synchronous
  readyOut : Outport  VectorParamsAs1DForOutWhenUnconnected=off
  wires:
  Logical Operator/1 -> readyOut/1
  frameSync/1 -> Delay/2
  readyIn/1 -> Logical Operator/1
  Delay/1 -> Logical Operator/2
  Constant/1 -> Delay/1

== system socmemlib/Memory Channel/Writer 1/To Memory Channel/Software Streaming To Memory Channel/Channel Streaming Slave Interface/MsgRecvCtrl ==
  Msg : Inport
  MsgRecvCtrl : TriggerPort  TriggerType=function-call  IsSimulinkFunction=on  FunctionName=MsgRecvCtrl  FunctionVisibility=scoped  VariantControl=(inherit)
  HWSW Message Receive : socsharedlib_internal/HWSW Message Receive  DataTypeStr=ChType  Dimensions=ChDimensions  QueueOverwriting=off  QueueLength=NumberOfBuffers  QueueLengthNum=8  QueueType=FIFO  InitialValue=[]  ValueSourceWhenQueueIsEmpty=Use initial value  MessageType=Stream  MessageID=HWSWMetadataID.Stream  SampleTime=-1  EnableDonePort=on  DiscardMessage=off
      settings: SourceProductBaseCode=HW
  Terminator : Terminator
  packToBytes : priv_hsblib_beta2/packToBytes  ChDimensions=ChDimensions  ChType=ChType  ChBitPacked=ChBitPacked  ChWidth=ChWidth  ChTDATAWidth=ChTDATAWidth  ChTDATAPadWidth=ChTDATAPadWidth  ChCompLength=ChCompLength  ChFrameGatherBufferSize=ChFrameGatherBufferSize  ChLength=ChLength
      settings: SourceProductBaseCode=HW
  packDataOut : ArgOut  DisableCoverage=on  OutDataTypeStr=uint8  PortDimensions=ChFrameGatherBufferSize  ArgumentName=packDataOut
  Valid : ArgOut  DisableCoverage=on  Port=2  OutDataTypeStr=boolean  ArgumentName=Valid
  data : Outport
  Done : Outport  Port=2
  wires:
  HWSW Message Receive/3 -> Valid/1
  packToBytes/1 -> packDataOut/1
  HWSW Message Receive/1 -> packToBytes/1, data/1
  HWSW Message Receive/4 -> Done/1
  HWSW Message Receive/2 -> Terminator/1
  Msg/1 -> HWSW Message Receive/1

== system socmemlib/Memory Channel/Writer 1/To Memory Channel/Software Streaming To Memory Channel/Channel Streaming Slave Interface/MsgReqCtrl ==
  MsgReqCtrl : TriggerPort  TriggerType=function-call  IsSimulinkFunction=on  FunctionName=MsgReqCtrl  FunctionVisibility=scoped  VariantControl=Variant
  Constant2 : Constant  OutDataTypeStr=uint32  SampleTime=-1
  Entity Generator : EntityGenerator  InputPortMessageModes=m  OutputPortMessageModes=m  GenerationMethod=Event-based  TimeSource=Signal port  Period=-1  GenerateAction=|  EntityType=Bus object  EntityTypeName=rteEvent
      | entity.name = [uint16('Dummy'), uint16(nan([1,64 - length('Dummy')]))]';
      | entity.type = uint32(5);
      | entity.index = uint32(0);
      settings: InputPortMap=u0
  Message Send : Send  OutputPortMessageModes=m
  Event : Outport  VectorParamsAs1DForOutWhenUnconnected=off
  wires:
  Message Send/1 -> Entity Generator/1
  Entity Generator/1 -> Event/1
  Constant2/1 -> Message Send/1
